simulink subsystem "consensusADMM"  (R2022b)
settings: Solver=VariableStepAuto  StartTime=0.0  StopTime=10.0  RelTol=1e-3
undefined symbols (not defined in the file): c
settings Model: Creator=is123  LastModifiedBy=is123

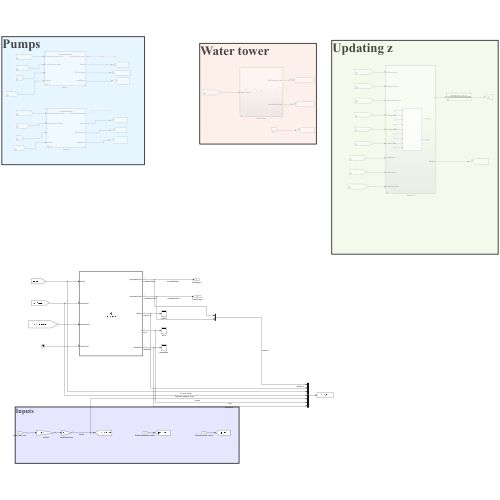
[thumbnail: Simulink's stored preview of the top-level diagram]
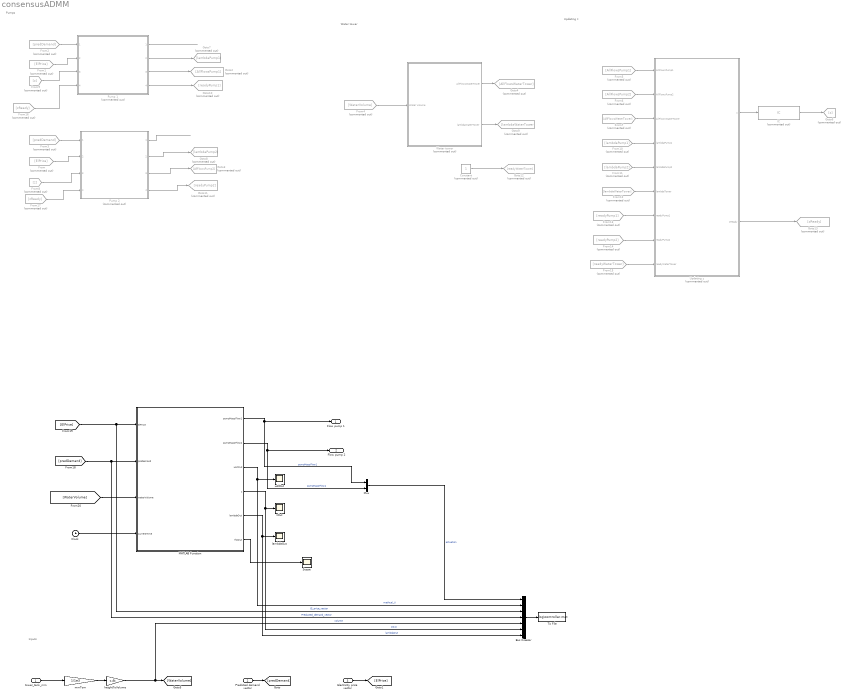
== system consensusADMM ==
  note: Updating z
  note: Water tower
  note: Pumps
  note: Inputs
  tower_tank_mm : Inport
  Predicted demand vector : Inport  Port=2
  Electricity price vector : Inport  Port=3
  Bus Creator : BusCreator  Inputs=7
  Clock : Clock
  Constant : Constant  Commented=on
  From : From  Commented=on  GotoTag=ElPrice
  From1 : From  Commented=on  GotoTag=ElPrice
  From10 : From  Commented=on  GotoTag=lambdaPump1
  From11 : From  Commented=on  GotoTag=lambdaPump2
  From12 : From  Commented=on  GotoTag=lambdaWaterTower
  From13 : From  Commented=on  GotoTag=readyPump1
  From14 : From  Commented=on  GotoTag=readyPump2
  From15 : From  Commented=on  GotoTag=readyWaterTower
  From16 : From  Commented=on  GotoTag=zReady
  From17 : From  Commented=on  GotoTag=zReady
  From2 : From  Commented=on  GotoTag=predDemand
  From3 : From  Commented=on  GotoTag=predDemand
  From4 : From  Commented=on  GotoTag=WaterVolume
  From5 : From  Commented=on  GotoTag=AllFlowsPump1
  From6 : From  Commented=on  GotoTag=AllFlowsPump2
  From7 : From  Commented=on  GotoTag=AllFlowsWaterTower
  From8 : From  Commented=on  GotoTag=z
  From9 : From  Commented=on  GotoTag=z
  Goto10 : Goto  Commented=on  GotoTag=readyPump1
  Goto11 : Goto  Commented=on  GotoTag=readyPump2
  Goto12 : Goto  Commented=on  GotoTag=readyWaterTower
  Goto13 : Goto  Commented=on  GotoTag=zReady
  Goto2 : Goto  Commented=on  GotoTag=AllFlowsPump1
  Goto3 : Goto  Commented=on  GotoTag=AllFlowsPump2
  Goto4 : Goto  Commented=on  GotoTag=AllFlowsWaterTower
  Goto6 : Goto  Commented=on  GotoTag=z
  Goto7 : Goto  Commented=on  GotoTag=lambdaPump1
  Goto8 : Goto  Commented=on  GotoTag=lambdaPump2
  Goto9 : Goto  Commented=on  GotoTag=lambdaWaterTower
  IC : InitialCondition  Commented=on  Value=zeros(c.Nu*c.Nc,1)
  MATLAB Function : MATLAB Function  TreatAsAtomicUnit=on  SystemSampleTime=600
  Mux : Mux  Inputs=2
  "Pump 1 " : Subsystem  Commented=on  ReferencedSubsystem=consensusPump  n_unit=1
  Pump 2 : Subsystem  Commented=on  ReferencedSubsystem=consensusPump  n_unit=2
  Scope : Scope
  To File : ToFile  Filename=log\controller.mat  MatrixName=ctrl  SaveFormat=Timeseries
  Updating z : Subsystem  Commented=on
  Water tower : Subsystem  Commented=on
  heightToVolume : Gain  Gain=c.At
  lambdaOut : Scope
  mmTom : Gain  Gain=1/1e3
  uAllOut : Scope
  zOut : Scope
  Flow pump 1 : Outport
  Flow pump 2 : Outport  Port=2
  wires:
  mmTom/1 -> heightToVolume/1
  tower_tank_mm/1 -> mmTom/1
  "Pump 1 "/1 -> ?
  Pump 2/1 -> ?
  Predicted demand vector/1 -> [predDemand]
  Electricity price vector/1 -> [ElPrice]
  From/1 -> Pump 2/2
  From1/1 -> "Pump 1 "/2
  From2/1 -> "Pump 1 "/1
  From3/1 -> Pump 2/1
  "Pump 1 "/3 -> Goto2/1
  Pump 2/3 -> Goto3/1
  Water tower/1(AllFlowsWaterTower) -> Goto4/1
  From4/1 -> Water tower/1(Water Volume)
  From5/1 -> Updating z/1(AllFlowsPump1)
  From6/1 -> Updating z/2(AllFlowsPump2)
  From7/1 -> Updating z/3(AllFlowsWaterTower)
  Updating z/1(z) -> IC/1
  From8/1 -> Pump 2/3
  From9/1 -> "Pump 1 "/3
  IC/1 -> Goto6/1
  From10/1 -> Updating z/4(lambdaPump1)
  "Pump 1 "/2 -> Goto7/1
  Pump 2/2 -> Goto8/1
  From11/1 -> Updating z/5(lambdaPump2)
  Water tower/2(lambdaWaterTower) -> Goto9/1
  From12/1 -> Updating z/6(lambdaTower)
  "Pump 1 "/4 -> Goto10/1
  Pump 2/4 -> Goto11/1
  From13/1 -> Updating z/7(readyPump1)
  From14/1 -> Updating z/8(readyPump2)
  From15/1 -> Updating z/9(readyWaterTower)
  Updating z/2(zReady) -> Goto13/1
  From16/1 -> "Pump 1 "/4
  From17/1 -> Pump 2/4
  Constant/1 -> Goto12/1
  [WaterVolume] -> MATLAB Function/3(waterVolume)
  MATLAB Function/2(pumpMassFlow2) -> Flow pump 2/1, Mux/2  "pumpMassFlow1"
  MATLAB Function/1(pumpMassFlow1) -> Flow pump 1/1, Mux/1  "pumpMassFlow1"
  MATLAB Function/4(z) -> zOut/1, Bus Creator/6  "zOut"
  MATLAB Function/5(lambdaOut) -> lambdaOut/1, Bus Creator/7  "lambdaOut"
  Bus Creator/1 -> To File/1
  heightToVolume/1 -> [WaterVolume], Bus Creator/5  "volume"
  [predDemand] -> Bus Creator/4, MATLAB Function/2(preDemand)  "Preducted_demand_vector"
  [ElPrice] -> Bus Creator/3, MATLAB Function/1(elPrice)  "El_price_vector"
  MATLAB Function/3(uAllOut) -> uAllOut/1, Bus Creator/2  "mathcal_U"
  Mux/1 -> Bus Creator/1  "actuation"
  Clock/1 -> MATLAB Function/4(currentTime)
  MATLAB Function/6(rhoOut) -> Scope/1

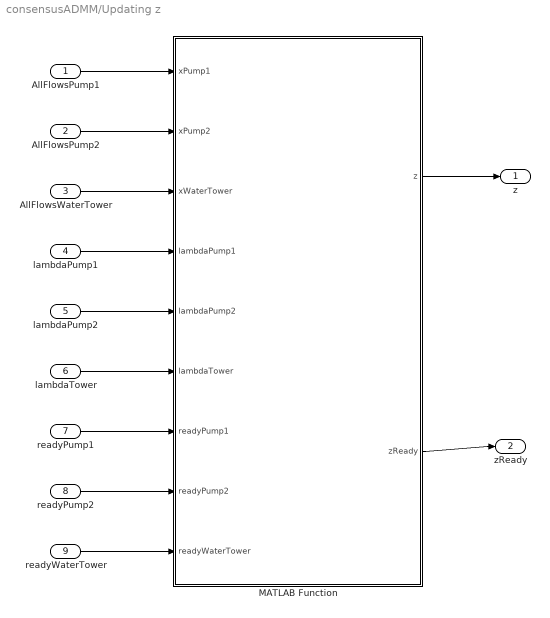
== system consensusADMM/Updating z ==
  AllFlowsPump1 : Inport
  AllFlowsPump2 : Inport  Port=2
  AllFlowsWaterTower : Inport  Port=3
  lambdaPump1 : Inport  Port=4
  lambdaPump2 : Inport  Port=5
  lambdaTower : Inport  Port=6
  readyPump1 : Inport  Port=7
  readyPump2 : Inport  Port=8
  readyWaterTower : Inport  Port=9
  MATLAB Function : MATLAB Function  TreatAsAtomicUnit=on  SystemSampleTime=3600/c.AccTime
  z : Outport
  zReady : Outport  Port=2
  wires:
  MATLAB Function/2(zReady) -> zReady/1
  readyWaterTower/1 -> MATLAB Function/9(readyWaterTower)
  readyPump2/1 -> MATLAB Function/8(readyPump2)
  readyPump1/1 -> MATLAB Function/7(readyPump1)
  lambdaTower/1 -> MATLAB Function/6(lambdaTower)
  lambdaPump2/1 -> MATLAB Function/5(lambdaPump2)
  lambdaPump1/1 -> MATLAB Function/4(lambdaPump1)
  AllFlowsWaterTower/1 -> MATLAB Function/3(xWaterTower)
  AllFlowsPump2/1 -> MATLAB Function/2(xPump2)
  AllFlowsPump1/1 -> MATLAB Function/1(xPump1)
  MATLAB Function/1(z) -> z/1

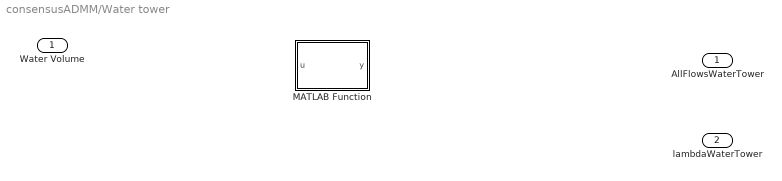
== system consensusADMM/Water tower ==
  Water Volume : Inport
  MATLAB Function : MATLAB Function  TreatAsAtomicUnit=on  SystemSampleTime=3600/c.AccTime
  AllFlowsWaterTower : Outport
  lambdaWaterTower : Outport  Port=2

== matlab function consensusADMM/MATLAB Function ==
  data: elPrice input; pumpMassFlow1 output; preDemand input; waterVolume input; pumpMassFlow2 output; uAllOut output; z output; lambdaOut output; currentTime input; rhoOut output
function [pumpMassFlow1, pumpMassFlow2, uAllOut,z,lambdaOut,rhoOut] = consensusADMM(elPrice,preDemand,waterVolume,currentTime)
    persistent z1 uAll rho
      c=scaled_standard_constants;  
    if isempty(z1) || isempty(uAll) ||isempty(rho)
        z1=zeros(c.Nu*c.Nc,1);
        uAll=zeros(c.Nu*c.Nc,c.Nu+1);
        rho=c.rho; 
    end
    xBar=zeros(c.Nu*c.Nc,c.iteration); 
rhoOut=rho; 
%Giving the system 10 minuts to start up!     
if currentTime < 200
        z=zeros(c.Nu*c.Nc,1);
        uAllOut=zeros(c.Nu*c.Nc,c.Nu+1);
        pumpMassFlow1=0; 
        pumpMassFlow2=0; 
        lambdaOut = zeros(c.Nc*c.Nu,c.Nu+1); 
else 
    
    % Updating inital geuss for consensus ADMM 
    x=zeros(c.Nc*c.Nu,c.Nu+1);
    x(:,1)=[uAll(c.Nu+1:end,1);uAll(end-c.Nu+1:end,1)]; 
    x(:,2)=[uAll(c.Nu+1:end,2);uAll(end-c.Nu+1:end,2)]; 
    x(:,3)=[uAll(c.Nu+1:end,3);uAll(end-c.Nu+1:end,3)];
    z=[z1(c.Nu+1:end,1);z1(end-c.Nu+1:end,1)];
    
    
    lambdaTilde=zeros(c.Nc*c.Nu,c.Nu+1); 
    lambda = zeros(c.Nc*c.Nu,c.Nu+1); 
    secretScaled=zeros(c.Nc*c.Nu,c.Nu+1); 
    
    yOut=zeros(c.Nu+1,c.Nc*c.Nu,c.Nu+1);
    yOutSum=zeros(c.Nc*c.Nu,1);
    
    %Saving demand and eletricty price in structure 
    data.Je=elPrice; 
    data.d=preDemand; 
    data.V=waterVolume; 

    
    
    %Setting up a few matrix needed for the consensus ADMM problem 
    data.A_1=zeros(c.Nc,c.Nu*c.Nc);
    index=1; 
    for i=1:c.Nc
        data.A_1(i,index:index+c.Nu-1) = 1;
        index=index+c.Nu;
    end
    
    %Lower trangiular matrix to add consumption and flows 
    data.A_2 = tril(ones(c.Nc,c.Nc));
    
    
    %Making vi vectors utilized to pick out 1 of the 3 pumps values, add them up
    %used to make extration limit. 
    data.v1=ones(c.Nu*c.Nc,1);
    data.v1(2:2:end) =0; 
    
    data.v2=ones(c.Nu*c.Nc,1);
    data.v2(1:2:end) =0;
    
    %Making matrix which picks out 1 of the pumps for the enitre control
    %horizion
    
    data.A_31=zeros(c.Nc,c.Nu*c.Nc);
    index=1; 
    for i=1:c.Nc
        data.A_31(i,index) = 1;
        index=index+c.Nu;
    end
    
    data.A_32=zeros(c.Nc,c.Nu*c.Nc);
    index=2; 
    for i=1:c.Nc
        data.A_32(i,index) = 1;
        index=index+c.Nu;
    end
        % Scaling the eletricity price if it is desired: 
    if c.scaledEletricityPrice == true
        data.Je=data.Je*0.4896/norm(data.Je); 
    end 
    
    tic 
    %% Going though the iterations: 
    for k=1:c.iteration
        x(:,1)=pump1(lambda(:,1),data,z,x(:,1),rho); 
        x(:,2)=pump2(lambda(:,2),data,z,x(:,2),rho);
        x(:,3)=WaterTower(lambda(:,3),data,z,x(:,3),rho);
    
        %Determine the z part for each of the pumps and making the function
        %output
        for index=1:c.Nu+1
            secretScaled(:,index)=c.scaling*(1/(c.Nu+1)*(x(:,index)+1/rho*lambda(:,index))+c.sMPCOffset);
            yOut(:,:,index)=generatedOutFromFunction(secretScaled(:,index));
        end 
        
        % Making the sum 
        yOutSum=yOut(:,:,1)+yOut(:,:,2)+yOut(:,:,3); 
        %Making rounding: 
        yOutSum=round(yOutSum); 
    
     a=GetFunctionParameter(yOutSum);
        
        %% Descaling it 
        %zTilde=(a)/c.scaling-((c.Nu+1)*c.sMPCOffset);
        %Updating z/updating consensus parameter 
        zTilde = sum(x,2)/(c.Nu+1) + 1/(rho*(c.Nu+1))*sum(lambda,2);
        %Updating lambda
        for i=1:c.Nu+1
            lambdaTilde(:,i) = lambda(:,i) + rho*(x(:,i)-z);
        end
            z = z - 1/(c.Nu+1+1)*(z-zTilde);
            lambda = lambda - 1/(c.Nu+1+1)*(lambda - lambdaTilde);
        
        %If rho should by varyed: 
        if c.varying_rho==true && k<c.varying_rho_iterations_numbers+1 
            %% Setting primal and dual residal to zero: 
            r=0;
            s=0; 
            xBar(:,k)=sum(x,2)/(c.Nu+1); 
                %Determining primal residual 
                disp("r:")
                for index=1:c.Nu+1 
                    r=norm(x(:,index)-xBar(:,k))+r
                end 
                
                %Determining dual residual 
                disp("s:")
                if k==1
                    s=sqrt((c.Nu+1)*rho^2*norm(xBar(:,k))^2)
                else
                    s=sqrt((c.Nu+1)*rho^2*norm(xBar(:,k)-xBar(:,k-1))^2)
                end 
                %Determine if the value of rho should change 
                 if r >c.mu*s 
                    rho=c.tauIncr*rho; 
                 elseif s>c.mu*r 
                     rho=rho/c.tauDecr; 
                 end 
                 disp("rho:")
                 rho 
       end  
       
       
    end %End for loop for iterations
    pumpMassFlow1=x(1,1);
    pumpMassFlow2=x(2,2);
    toc
        uAllOut=x; 
        rhoOut=rho; 
    lambdaOut=lambda; 
end %End if statement
    
    

    

end %end function

== matlab function consensusADMM/Updating z/MATLAB Function ==
  data: xPump1 input; xPump2 input; z output; xWaterTower input; lambdaPump1 input; lambdaPump2 input; lambdaTower input; zReady output; readyPump1 input; readyPump2 input; readyWaterTower input
function [z,zReady] = updateZ(xPump1,xPump2,xWaterTower,lambdaPump1,lambdaPump2,lambdaTower,readyPump1,readyPump2,readyWaterTower)
%Here it is desired to determine the next value of z, 
%Loading in standard contants
c=scaled_standard_constants; 

%Defining the size of the output
z=zeros(c.Nu*c.Nc,1); 

for k=1:c.iteration
    zReady=0; 
    %Waiting for the agents to be ready 
    while readyPump1 == 0 || readyPump2== 0 ||readyWaterTower== 0 
    
    end 
    %Making is of the term in the sum: 
    zPump1=1/c.Nu*(xPump1+1/c.rho*lambdaPump1); 
    
    zPump2=1/c.Nu*(xPump2+1/c.rho*lambdaPump2);
    
    %zWaterTower=1/c.Nu*(xWaterTower+1/c.rho*lambdaTower);
    
    %Addning them up to get the output:
    z=zPump1+zPump2;%+zWaterTower;
    zReady=1; 
    %Giving the other a chance to see that a new z is ready!  
    pause(0.05); 

end

== matlab function consensusADMM/Water tower/MATLAB Function ==
  data: u input; y output
function y = fcn(u)

y = u;
